simulink model "simulink_caso4"  (R2023a)
settings: Solver=VariableStepAuto  StartTime=0.0  StopTime=10.0  RelTol=1e-3
undefined symbols (not defined in the file): A, Aest, B, Best, C, Cest, D, Dest, K, K00
libraries: simulink x1
settings Model: Creator=Agustin  LastModifiedBy=Agustin

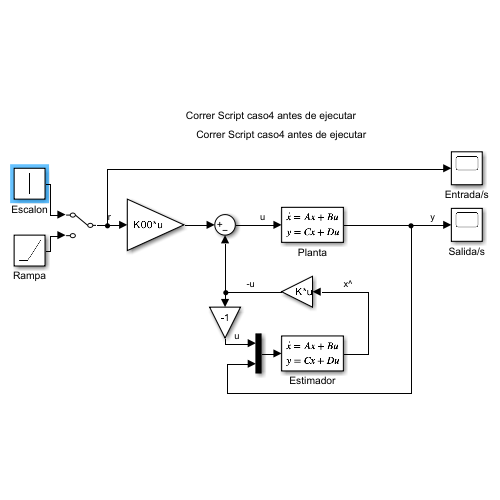
[thumbnail: Simulink's stored preview of the top-level diagram]
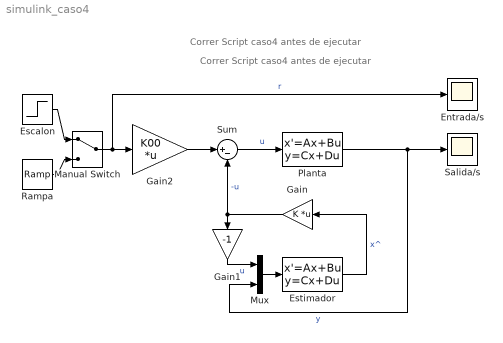
== system simulink_caso4 ==
  note: Correr Script caso4 antes de ejecutar
  note: Correr Script caso4 antes de ejecutar
  Entrada/s : Scope
  Escalon : Step  SampleTime=0
  Estimador : StateSpace  A=Aest  B=Best  C=Cest  D=Dest  InitialCondition=0
  Gain : Gain  Gain=K  Multiplication=Matrix(K*u)
  Gain1 : Gain  Gain=-1
  Gain2 : Gain  Gain=K00  Multiplication=Matrix(K*u)
  Manual Switch : ManualSwitch
  Mux : Mux  Inputs=2
  Planta : StateSpace  A=A  B=B  C=C  D=D  InitialCondition=0
  Rampa : simulink/Sources/Ramp  slope=1  start=0  InitialOutput=0
  Salida/s : Scope
  Sum : Sum  Inputs=|+-
  wires:
  Estimador/1 -> Gain/1  "x^"
  Sum/1 -> Planta/1  "u"
  Planta/1 -> Mux/2, Salida/s/1  "y"
  Manual Switch/1 -> Entrada/s/1, Gain2/1  "r"
  Mux/1 -> Estimador/1
  Gain/1 -> Gain1/1, Sum/2  "-u"
  Gain2/1 -> Sum/1
  Gain1/1 -> Mux/1  "u"
  Escalon/1 -> Manual Switch/1
  Rampa/1 -> Manual Switch/2
